simulink library "motohawk_engine_motoshare_lib"  (Simulink 6.3)
undefined symbols (not defined in the file or in its folder): cast_val, IndPowerMax, lookup_group, motohawk_tex, motohawk_vardec_config_group, motohawk_vardec_path, SampleTime, SteadyStateECT, txtTitle, WarmUpTimeConst
libraries: MotoHawk_lib x211, motohawk_control_primitives_lib x20, motohawk_annotations_lib x7, motohawk_engine_lib x5, AutoDoc_lib x4, motohawk_control_primitives_lib_new x3, motohawk_control_primitives_motoshare_lib x2
(part 7 of 7)

== system motohawk_engine_motoshare_lib/Linear Sensor Characterization w Adapt/AdaptPoints/High Side Adapt ==
  AdaptRequest : Inport
  AdaptEnable : Inport  Port=2
  CurAdaptPt : Inport  Port=3
  AdaptRangeMax : Inport  Port=4
  AdaptRangeMin : Inport  Port=5
  AdaptMinDelta : Inport  Port=6
  MaxLast5 : Inport  Port=7
  Abs : Abs  SaturateOnIntegerOverflow=on
  Data Type Conversion : DataTypeConversion  OutDataTypeMode=double  SaturateOnIntegerOverflow=on  RndMeth=Zero
  Logical Operator1 : Logic  Inputs=5  AllPortsSameDT=off
  Logical Operator2 : Logic  Operator=OR  AllPortsSameDT=off
  Logical Operator4 : Logic  Inputs=4  AllPortsSameDT=off
  Relational Operator3 : RelationalOperator  Operator=>  LogicOutDataTypeMode=Boolean
  Relational Operator5 : RelationalOperator  Operator=<=  LogicOutDataTypeMode=Boolean
  Relational Operator6 : RelationalOperator  LogicOutDataTypeMode=Boolean
  Relational Operator9 : RelationalOperator  Operator=>  LogicOutDataTypeMode=Boolean
  Store Current Position : Subsystem  TreatAsAtomicUnit=on
  Sum2 : Sum  Inputs=|+-  SaturateOnIntegerOverflow=on
  AdaptedEndPt : Outport
  wires:
  Logical Operator2/1 -> Store Current Position/Enable
  Logical Operator1/1 -> Logical Operator2/1
  AdaptRangeMin/1 -> Relational Operator6/2
  AdaptRangeMax/1 -> Relational Operator5/2
  Relational Operator6/1 -> Logical Operator1/3, Logical Operator4/2
  Relational Operator5/1 -> Logical Operator1/2, Logical Operator4/1
  Relational Operator9/1 -> Logical Operator1/1
  CurAdaptPt/1 -> Data Type Conversion/1
  Sum2/1 -> Abs/1
  Relational Operator3/1 -> Logical Operator1/5
  Abs/1 -> Relational Operator3/1
  AdaptMinDelta/1 -> Relational Operator3/2
  Data Type Conversion/1 -> AdaptedEndPt/1, Relational Operator9/2, Sum2/2
  AdaptEnable/1 -> Logical Operator1/4, Logical Operator4/3
  MaxLast5/1 -> Sum2/1, Store Current Position/1(In), Relational Operator9/1, Relational Operator5/1, Relational Operator6/1
  Logical Operator4/1 -> Logical Operator2/2
  AdaptRequest/1 -> Logical Operator4/4

== system motohawk_engine_motoshare_lib/Linear Sensor Characterization w Adapt/AdaptPoints/Low Side Adapt ==
  AdaptRequest : Inport
  AdaptEnable : Inport  Port=2
  CurAdaptPt : Inport  Port=3
  AdaptRangeMax : Inport  Port=4
  AdaptRangeMin : Inport  Port=5
  AdaptMinDelta : Inport  Port=6
  MaxLast5 : Inport  Port=7
  Abs : Abs  SaturateOnIntegerOverflow=on
  Data Type Conversion : DataTypeConversion  OutDataTypeMode=double  SaturateOnIntegerOverflow=on  RndMeth=Zero
  Logical Operator1 : Logic  Inputs=5  AllPortsSameDT=off
  Logical Operator2 : Logic  Operator=OR  AllPortsSameDT=off
  Logical Operator4 : Logic  Inputs=4  AllPortsSameDT=off
  Relational Operator3 : RelationalOperator  Operator=>  LogicOutDataTypeMode=Boolean
  Relational Operator5 : RelationalOperator  Operator=<=  LogicOutDataTypeMode=Boolean
  Relational Operator6 : RelationalOperator  LogicOutDataTypeMode=Boolean
  Relational Operator9 : RelationalOperator  Operator=<  LogicOutDataTypeMode=Boolean
  Store Current Position : Subsystem  TreatAsAtomicUnit=on
  Sum2 : Sum  Inputs=|+-  SaturateOnIntegerOverflow=on
  AdaptedEndPt : Outport
  wires:
  MaxLast5/1 -> Relational Operator6/1, Relational Operator5/1, Relational Operator9/1, Store Current Position/1(In), Sum2/1
  AdaptEnable/1 -> Logical Operator1/4, Logical Operator4/3
  Data Type Conversion/1 -> Sum2/2, Relational Operator9/2, AdaptedEndPt/1
  AdaptMinDelta/1 -> Relational Operator3/2
  Abs/1 -> Relational Operator3/1
  Relational Operator3/1 -> Logical Operator1/5
  Sum2/1 -> Abs/1
  CurAdaptPt/1 -> Data Type Conversion/1
  Relational Operator9/1 -> Logical Operator1/1
  Relational Operator5/1 -> Logical Operator1/2, Logical Operator4/1
  Relational Operator6/1 -> Logical Operator1/3, Logical Operator4/2
  AdaptRangeMax/1 -> Relational Operator5/2
  AdaptRangeMin/1 -> Relational Operator6/2
  Logical Operator1/1 -> Logical Operator2/1
  Logical Operator2/1 -> Store Current Position/Enable
  AdaptRequest/1 -> Logical Operator4/4
  Logical Operator4/1 -> Logical Operator2/2

== system motohawk_engine_motoshare_lib/Linear Sensor Characterization w Adapt/AdaptPoints/MinMaxFilter ==
  Input : Inport
  Bus Creator : BusCreator  Inputs=2
  MinMax : MinMax  Function=max  Inputs=5  SaturateOnIntegerOverflow=on  InputSameDT=on
  MinMax1 : MinMax  Inputs=5  SaturateOnIntegerOverflow=on  InputSameDT=on
  Unit Delay{,1,3..4} (4 alike) : UnitDelay  SampleTime=-1
  Min_Max : Outport
  wires:
  Bus Creator/1 -> Min_Max/1
  Unit Delay4/1 -> MinMax/2, MinMax1/4, Unit Delay3/1
  Unit Delay3/1 -> MinMax/3, MinMax1/3, Unit Delay/1
  Unit Delay/1 -> MinMax/4, Unit Delay1/1, MinMax1/2
  Unit Delay1/1 -> MinMax/5, MinMax1/1
  MinMax/1 -> Bus Creator/1  "max_last5"
  MinMax1/1 -> Bus Creator/2  "min_last5"
  Input/1 -> MinMax1/5, MinMax/1, Unit Delay4/1

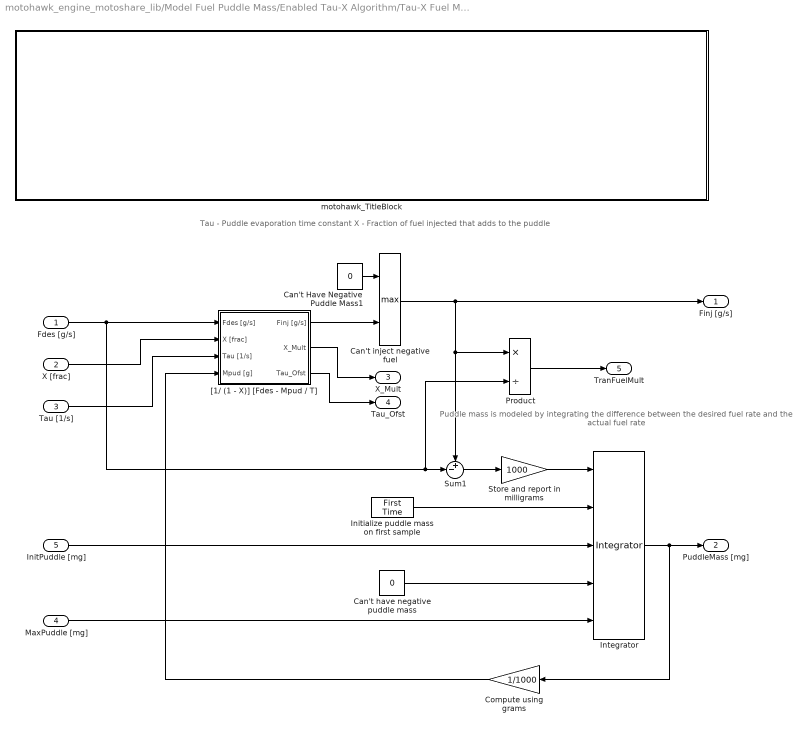
== system motohawk_engine_motoshare_lib/Model Fuel Puddle Mass/Enabled Tau-X Algorithm/Tau-X Fuel Model ==
  note: Tau - Puddle evaporation time constant
      | X - Fraction of fuel injected that adds to the puddle
  note: Puddle mass is modeled by integrating
      | the difference between the desired fuel rate
      | and the actual fuel rate
  Fdes [g/s] : Inport
  X [frac] : Inport  Port=2
  Tau [1/s] : Inport  Port=3
  MaxPuddle [mg] : Inport  Port=4
  InitPuddle [mg] : Inport  Port=5
  Can't Have Negative Puddle Mass1 : Constant  Value=0
  Can't have negative puddle mass : Constant  Value=0
  Can't inject negative fuel : MinMax  Function=max  Inputs=2  SaturateOnIntegerOverflow=on  InputSameDT=on
  Compute using grams : Gain  Orientation=left  Gain=1/1000  SaturateOnIntegerOverflow=on
  Initialize puddle mass on first sample : motohawk_control_primitives_lib/First Time
  Integrator : motohawk_control_primitives_lib/Integrator  samp_time=samp_time
  Product : Product  Inputs=*/  SaturateOnIntegerOverflow=on
  Store and report in milligrams : Gain  Gain=1000  SaturateOnIntegerOverflow=on
  Sum1 : Sum  Inputs=+-|  SaturateOnIntegerOverflow=on  InputSameDT=on
  "[1/ (1 - X)] [Fdes - Mpud / T]" : Subsystem
  motohawk_TitleBlock : Subsystem  mask{BlockType_='Mototron_Title_Block', ttl='Tau-X Transient Fueling Model\newline\rmUse parameters Tau and X to predictively model a fuel puddle mass\newlineTake into account evaporation from the puddle when calculating the fuel to inject,\newlineso that transient changes in fueling rate do not cause overly lean or rich burns', im=mh.jpg}
      mask prompts: ttl "Description"; im "Image FIle"
      mask init:
      | set_param(gcb,'BlockType_','''Mototron_Title_Block''')
      | set_param(gcb,'MaskVisibilityString','off,on,on');
      mask Display:
      | image(imread(im),[0.31 0.66 0.31 0.35])
      | 
      | plot([0 0 1 1 0],[0 1 1 0 0])
      | plot([.3 1],[0.65 0.65])
      | plot([.3 .3],[0.1 1.0])
      | plot([0 1],[0.1 0.1])
      | plot([0.91 0.91],[0 0.1])
      | text(1,1,'\fontsize{22}\it\fontname{Arial Black}MotoTron Corporation \fontname{Arial}\fontsize{10}\newline505 Marion Road, Oshkosh, WI, 54901\newlinewww.mototron.com (734) 822-7700','verticalAlignment','Top','horizontalAlignment','Right','texmode','on')
      | text(0.01,1,['\fontsize{14}\it\bfPROPRIETARY\newlineAND CONFIDENTIAL\newline\fontsize{10}
      | THE INFORMATION CONTAINED IN THIS\newline
      | DRAWING IS THE SOLE PROPERTY OF\newline
      | MOTOTRON.  ANY REPRODUCTION IN\newline
      | PART OR AS A WHOLE WITHOUT THE\newline
      | WRITTEN PERMISSION OF MOTOTRON\newline
      | IS PROHIBITED.\fontsize{16}\rm\copyright\rm\fontsize{10} 2004' ],'verticalAlignment','Top','horizontalAlignment','Left','texmode','on')
      | 
      | text(0.9,0,['\fontsize{11}\bfPath: \rm' strrep(motohawk_vardec_path(gcb),'_','\_')],'verticalAlignment','Bottom','horizontalAlignment','Right','texmode','on')
      | text(0.31,0.65,['\fontsize{10}\bfDescription:'],'verticalAlignment','Top','horizontalAlignment','Left','texmode','on')
      | 
      | text(0.31,0.55,['\fontsize{14}\bf' ttl],'verticalAlignment','Top','horizontalAlignment','Left','texmode','on')
      | text(0.99,0,['\fontsize{11}\bfREV: \rm' motohawk_build_version],'verticalAlignment','Bottom','horizontalAlignment','Right','texmode','on')
  Finj [g/s] : Outport
  PuddleMass [mg] : Outport  Port=2
  X_Mult : Outport  Port=3
  Tau_Ofst : Outport  Port=4
  TranFuelMult : Outport  Port=5
  wires:
  Product/1 -> TranFuelMult/1
  "[1/ (1 - X)] [Fdes - Mpud / T]"/3(Tau_Ofst) -> Tau_Ofst/1
  "[1/ (1 - X)] [Fdes - Mpud / T]"/2(X_Mult) -> X_Mult/1
  Can't Have Negative Puddle Mass1/1 -> Can't inject negative fuel/1
  Can't inject negative fuel/1 -> Product/1, Sum1/1, Finj [g/s]/1
  "[1/ (1 - X)] [Fdes - Mpud / T]"/1(Finj [g/s]) -> Can't inject negative fuel/2
  InitPuddle [mg]/1 -> Integrator/3
  Initialize puddle mass on first sample/1 -> Integrator/2
  Can't have negative puddle mass/1 -> Integrator/4
  MaxPuddle [mg]/1 -> Integrator/5
  Integrator/1 -> PuddleMass [mg]/1, Compute using grams/1
  Sum1/1 -> Store and report in milligrams/1
  X [frac]/1 -> "[1/ (1 - X)] [Fdes - Mpud / T]"/2(X [frac])
  Tau [1/s]/1 -> "[1/ (1 - X)] [Fdes - Mpud / T]"/3(Tau [1/s])
  Fdes [g/s]/1 -> Product/2, Sum1/2, "[1/ (1 - X)] [Fdes - Mpud / T]"/1(Fdes [g/s])
  Compute using grams/1 -> "[1/ (1 - X)] [Fdes - Mpud / T]"/4(Mpud [g])
  Store and report in milligrams/1 -> Integrator/1

== system motohawk_engine_motoshare_lib/Model Fuel Puddle Mass/Enabled Tau-X Algorithm/motohawk_TitleBlock ==

== system motohawk_engine_motoshare_lib/Normalized Effective Combustion Chamber Temperature/Integrate an offset to ECT  Reset offset when engine is stopped./Integrator ==
  note: Discrete Integrator,
      | with output and state saturation.
  In : Inport  Orientation=left
  Rst : Inport  Port=2
  IC : Inport  Port=3
  Min : Inport  Orientation=left  Port=4
  Max : Inport  Orientation=left  Port=5
  Data Type Conversion : DataTypeConversion  RndMeth=Zero
  Product : Product  Orientation=left  SaturateOnIntegerOverflow=on  InputSameDT=on
  Saturation : Subsystem  Orientation=left  mask(Saturation){}
      mask help: Saturation block.
      mask Display:
      | patch([0 0 1 1], [0 0.075 0.075 0], [230/255 0/255 0/255])
      | patch([0 0 1 1], [0.025 0.05 0.05 0.025], [150/255 0/255 0/255])
      | patch([0 0 1 1], [0 0.025 0.025 0], [0/255 0/255 0/255])
      | 
      | plot([.2 .4 .6 .8], [.2 .2 .9 .9])
  Sum : Sum  Orientation=left  Inputs=++|  SaturateOnIntegerOverflow=on  InputSameDT=on
  Switch1 : Switch  Threshold=1  ZeroCross=off  SaturateOnIntegerOverflow=on  InputSameDT=on
  Unit Delay : UnitDelay  Orientation=left  SampleTime=-1
  motohawk_delta_time : S-Function  Orientation=left  FunctionName=motohawk_sfun_delta_time  Parameters=samp_time, double(init_val)  mask(MotoHawk Delta Time){samp_time=samp_time, init_val=0}
      mask prompts: samp_time "Sample Time"; init_val "Initial Value"
      mask help:
      | Outputs the delta time since the last time this block was called (in seconds).
      |
      | If a positive 'Sample Time' is entered, this constant value will be output every time.  The output data type will be the same as the 'Sample Time' parameter.  In this case, the 'Initial Value' parameter is unused.
      |
      | If a zero or negative 'Sample Time' is entered, the block will calculate the delta time, and the block\ will output 'Initial Value' the first time it is called.
      |
      | Using a constant sample time is more efficient than an inherited sample time, because it does not generate extra code and RAM to dynamically calculate the delta time.
      |
      | Note that the block still runs with inherited sample-time in the Simulink environment, regardless of what is entered.  It is legal to insert a 'wrong' value into the Sample Time (a value that doesn't actually represent the number of seconds between executions), and the block will happily output that value.
      |
      | ---------------------------------------------------------------------
      | Copyright 2004 MotoTron, Inc.  All Rights Reserved.
      mask Display:
      | patch([0 0 1 1], [0 1 1 0], [220/255 220/255 220/255])
      | patch([0 0 1 1], [0 0.075 0.075 0], [230/255 0/255 0/255])
      | patch([0 0 1 1], [0.025 0.05 0.05 0.025], [150/255 0/255 0/255])
      | patch([0 0 1 1], [0 0.025 0.025 0], [0/255 0/255 0/255])
      | 
      | disp('dT');
  Out : Outport
  wires:
  IC/1 -> Switch1/1
  Max/1 -> Saturation/3(max)
  Min/1 -> Saturation/2(min)
  Data Type Conversion/1 -> Switch1/2
  Rst/1 -> Data Type Conversion/1
  Unit Delay/1 -> Switch1/3
  Product/1 -> Sum/2
  In/1 -> Product/1
  motohawk_delta_time/1 -> Product/2
  Switch1/1 -> Out/1, Sum/1
  Sum/1 -> Saturation/1(in)
  Saturation/1(out) -> Unit Delay/1

== system motohawk_engine_motoshare_lib/O2A/Equivalence Ratio Perturbation/Hysteresis ==
  note: Hi & !Lo => Hi
      | Lo & !Hi => Lo
      | Otherwise, Hold
  Hi : Inport
  Lo : Inport  Port=2
  Combinatorial  Logic : CombinatorialLogic  TruthTable=[0 0;0 1;1 1;0 0]
  Demux : Demux  Outputs=2
  Mux : Mux  Inputs=2
  Switch1 : Switch  Threshold=0.5  SaturateOnIntegerOverflow=on  InputSameDT=on
  Unit Delay : UnitDelay  Orientation=left  SampleTime=-1
  "Out (Lo=0, Hi=1)" : Outport
  wires:
  Lo/1 -> Mux/2
  Hi/1 -> Mux/1
  Switch1/1 -> "Out (Lo=0, Hi=1)"/1, Unit Delay/1
  Unit Delay/1 -> Switch1/3
  Demux/2 -> Switch1/2
  Demux/1 -> Switch1/1
  Combinatorial  Logic/1 -> Demux/1
  Mux/1 -> Combinatorial  Logic/1

== system motohawk_engine_motoshare_lib/Speed Density - MAP Referenced - Adaptive/Adapt Volumetric Efficiency/Adapt VolEff Map ==
  Error : Inport
  AdaptEnabled : Inport  Port=2
  VE : Inport  Port=3
  Enable : EnablePort
  Logical Operator : Logic  AllPortsSameDT=off  OutDataTypeMode=Boolean
  Logical Operator1 : Logic  AllPortsSameDT=off  OutDataTypeMode=Boolean
  Relational Operator1 : RelationalOperator  Operator=<=  LogicOutDataTypeMode=Boolean
  Relational Operator2 : RelationalOperator  LogicOutDataTypeMode=Boolean
  motohawk_adapt_table : MotoHawk_lib/Lookup Tables/motohawk_adapt_table  nam='VolEff'  typ=double  mode=Adapt between points
  motohawk_calibration1 : MotoHawk_lib/Calibration & Probing Blocks/motohawk_calibration  nam='VEAdaptMax'  val=1  storage=Calibration  show_more=on  name_source=Use Parameter  data_type=Inherit from 'Default Value'  read_level=1  write_level=1  ovr_cals=on  view_as=Number  enum_struct={'Disabled', 'Enabled'}  vector_style=Wide Row  use_help_units=on  help='Maximum value that can be adapted into the VE table.'  units=''  use_header_enum=off  row_header_enum={}  col_header_enum={}  use_min_max=on  min_val=0  max_val=1  use_precision=off  precision='8.6'  gain=1  offset=0  exp=1  use_mototune_group=on  mototune_group=lookup_group(gcb)
  motohawk_calibration2 : MotoHawk_lib/Calibration & Probing Blocks/motohawk_calibration  nam='VEAdaptMin'  val=0  storage=Calibration  show_more=on  name_source=Use Parameter  data_type=Inherit from 'Default Value'  read_level=1  write_level=1  ovr_cals=on  view_as=Number  enum_struct={'Disabled', 'Enabled'}  vector_style=Wide Row  use_help_units=on  help='Minimum value that can be adapted into the VE table.'  units=''  use_header_enum=off  row_header_enum={}  col_header_enum={}  use_min_max=on  min_val=-inf  max_val=inf  use_precision=off  precision='8.6'  gain=1  offset=0  exp=1  use_mototune_group=on  mototune_group=lookup_group(gcb)
  motohawk_fault_def : MotoHawk_lib/Fault Management Blocks/motohawk_fault_def  nam='VEAdaptRangeHi'  mode=Enabled  id=[]  x=25  y=50  input_suspected=on  indeterminate=off  increment_xy=on  downsample_count=1  ovr_cals=on  ovr_actions=on  show_actions=off  action1_name=''  action1_cond=(None)  action2_name=''  action2_cond=(None)  action3_name=''  action3_cond=(None)  action4_name=''  action4_cond=(None)
  motohawk_fault_def1 : MotoHawk_lib/Fault Management Blocks/motohawk_fault_def  nam='VEAdaptRangeLow'  mode=Enabled  id=[]  x=25  y=50  input_suspected=on  indeterminate=off  increment_xy=on  downsample_count=1  ovr_cals=on  ovr_actions=on  show_actions=off  action1_name=''  action1_cond=(None)  action2_name=''  action2_cond=(None)  action3_name=''  action3_cond=(None)  action4_name=''  action4_cond=(None)
  wires:
  Error/1 -> motohawk_adapt_table/1
  motohawk_calibration2/1 -> motohawk_adapt_table/2, Relational Operator1/2
  motohawk_calibration1/1 -> motohawk_adapt_table/3, Relational Operator2/2
  Relational Operator2/1 -> Logical Operator1/1
  Relational Operator1/1 -> Logical Operator/1
  Logical Operator1/1 -> motohawk_fault_def/1
  Logical Operator/1 -> motohawk_fault_def1/1
  VE/1 -> Relational Operator1/1, Relational Operator2/1
  AdaptEnabled/1 -> Logical Operator1/2, Logical Operator/2

== system motohawk_engine_motoshare_lib/Speed Density - MAP Referenced - Adaptive/Adapt Volumetric Efficiency/Safe Divide ==
  X : Inport
  Inport : Inport  Port=2
  Constant : Constant  Value=0
  Relational Operator : RelationalOperator  Operator=~=  ZeroCross=off  InputSameDT=on
  Subsystem : Subsystem
  " " : Outport  InitialOutput=0
  wires:
  Constant/1 -> Relational Operator/1
  Relational Operator/1 -> Subsystem/Enable
  Subsystem/1(Out1) -> " "/1
  ? -> Relational Operator/2, Subsystem/2(In2)
  X/1 -> Subsystem/1(In1)

== system motohawk_engine_motoshare_lib/Linear Sensor Characterization w Adapt/AdaptPoints/High Side Adapt/Store Current Position ==
  In : Inport
  Enable : EnablePort
  Data Type Conversion2 : DataTypeConversion  OutDataTypeMode=uint16  SaturateOnIntegerOverflow=on  RndMeth=Zero
  motohawk_data_write : MotoHawk_lib/Data Storage Blocks/motohawk_data_write  source=Lookup By Name  structure=Scalar  operation=Write entire data structure at once  sz_vec=-1  sz_row=3  sz_col=2  typ=uint16  nam=[prefix 'RawAdptHi']  checkNull=off  write_read_only=off  struct_inst_name='Struct1'
  wires:
  Data Type Conversion2/1 -> motohawk_data_write/1
  In/1 -> Data Type Conversion2/1

== system motohawk_engine_motoshare_lib/Linear Sensor Characterization w Adapt/AdaptPoints/Low Side Adapt/Store Current Position ==
  In : Inport
  Enable : EnablePort
  Data Type Conversion2 : DataTypeConversion  OutDataTypeMode=uint16  SaturateOnIntegerOverflow=on  RndMeth=Zero
  motohawk_data_write : MotoHawk_lib/Data Storage Blocks/motohawk_data_write  source=Lookup By Name  structure=Scalar  operation=Write entire data structure at once  sz_vec=-1  sz_row=3  sz_col=2  typ=uint16  nam=[prefix 'RawAdptLow']  checkNull=off  write_read_only=off  struct_inst_name='Struct1'
  wires:
  In/1 -> Data Type Conversion2/1
  Data Type Conversion2/1 -> motohawk_data_write/1

== system motohawk_engine_motoshare_lib/Model Fuel Puddle Mass/Enabled Tau-X Algorithm/Tau-X Fuel Model/[1/ (1 - X)] [Fdes - Mpud / T] ==
  Fdes [g/s] : Inport
  X [frac] : Inport  Port=2
  Tau [1/s] : Inport  Port=3
  Mpud [g] : Inport  Port=4
  Constant : Constant
  Product : Product  Inputs=*/  SaturateOnIntegerOverflow=on  InputSameDT=on
  Product1 : Product  Inputs=**  SaturateOnIntegerOverflow=on  InputSameDT=on
  Product2 : Product  Inputs=*/  SaturateOnIntegerOverflow=on  InputSameDT=on
  Sum : Sum  Inputs=|+-  SaturateOnIntegerOverflow=on  InputSameDT=on
  Sum1 : Sum  Inputs=|+-  SaturateOnIntegerOverflow=on  InputSameDT=on
  Finj [g/s] : Outport
  X_Mult : Outport  Port=2
  Tau_Ofst : Outport  Port=3
  wires:
  Constant/1 -> Product/1, Sum/1
  X [frac]/1 -> Sum/2
  Sum/1 -> Product/2
  Mpud [g]/1 -> Product2/1
  Tau [1/s]/1 -> Product2/2
  Fdes [g/s]/1 -> Sum1/1
  Product2/1 -> Tau_Ofst/1, Sum1/2
  Sum1/1 -> Product1/1  "Fdes - Mpud / T"
  Product/1 -> X_Mult/1, Product1/2  "1 / (1 - X)"
  Product1/1 -> Finj [g/s]/1

== system motohawk_engine_motoshare_lib/Model Fuel Puddle Mass/Enabled Tau-X Algorithm/Tau-X Fuel Model/motohawk_TitleBlock ==

== system motohawk_engine_motoshare_lib/Normalized Effective Combustion Chamber Temperature/Integrate an offset to ECT  Reset offset when engine is stopped./Integrator/Saturation ==
  note: Output 'In' when between Min and Max,
      | and saturate against limits otherwise.
  in : Inport
  min : Inport  Port=2
  max : Inport  Port=3
  MinMax : MinMax  Function=max  Inputs=2  ZeroCross=off  SaturateOnIntegerOverflow=on  InputSameDT=on
  MinMax1 : MinMax  Inputs=2  ZeroCross=off  SaturateOnIntegerOverflow=on  InputSameDT=on
  out : Outport
  wires:
  MinMax1/1 -> out/1
  max/1 -> MinMax1/2
  min/1 -> MinMax/2
  in/1 -> MinMax/1
  MinMax/1 -> MinMax1/1

== system motohawk_engine_motoshare_lib/Speed Density - MAP Referenced - Adaptive/Adapt Volumetric Efficiency/Safe Divide/Subsystem ==
  In1 : Inport
  In2 : Inport  Port=2
  Enable : EnablePort
  Product1 : Product  Inputs=*/  SaturateOnIntegerOverflow=on  InputSameDT=on
  Out1 : Outport  InitialOutput=0
  wires:
  In2/1 -> Product1/2
  Product1/1 -> Out1/1
  In1/1 -> Product1/1

== stateflow chart Idle Governor/Idle State Determination/Idle State Machine ==
  state OffIdle
    /en: IdleState = 3;
  state Flaring
    /en: IdleState = 1;
  state OnIdle
    /en: IdleState = 2;
  (default) -> Flaring
  Flaring -> OffIdle [order 1] : [ThrPosHigh || !IdleEnable]
  OffIdle -> OnIdle : [RPMLow && ThrPosLow && IdleEnable]
  Flaring -> OnIdle [order 2] : [RPMFalling && ThrPosLow]
  OnIdle -> OffIdle : [ThrPosHigh || !IdleEnable]
  data: IdleEnable input boolean; RPMFalling input boolean; RPMLow input boolean; ThrPosLow input boolean; ThrPosHigh input boolean; IdleState output uint8
